simulink library "ECEF2LLA"  (R2018b)
settings: Solver=VariableStepAuto  StartTime=0.0  StopTime=10.0  RelTol=1e-3
settings Model: Creator=BI28030  LastModifiedBy=BI28030

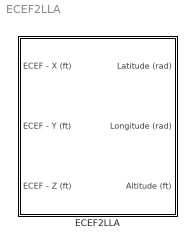
== system ECEF2LLA ==
  ECEF2LLA : Subsystem  mask{a=6378137, b=6356752.31424518}
      mask prompts: a "Semi-major axis (meters)"; b "Semi-major axis (meters)"

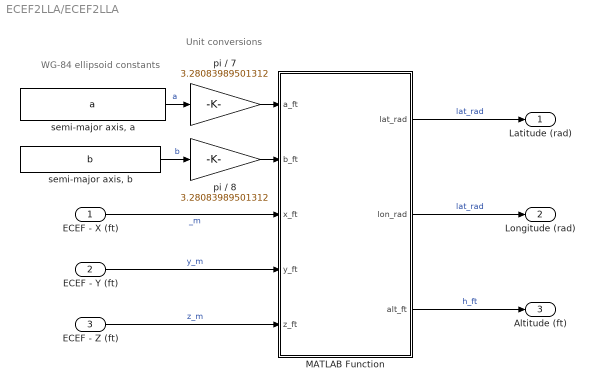
== system ECEF2LLA/ECEF2LLA ==
  note: WG-84 ellipsoid constants
  note: Unit conversions
  ECEF - X (ft) : Inport
  ECEF - Y (ft) : Inport  Port=2
  ECEF - Z (ft) : Inport  Port=3
  MATLAB Function : MATLAB Function  TreatAsAtomicUnit=on
  pi / 7 : Gain  Gain=3.28083989501312
  pi / 8 : Gain  Gain=3.28083989501312
  "semi-major axis, a" : Constant  Value=a
  "semi-major axis, b" : Constant  Value=b
  Latitude (rad) : Outport
  Longitude (rad) : Outport  Port=2
  Altitude (ft) : Outport  Port=3
  wires:
  pi / 8/1 -> MATLAB Function/2(b_ft)
  pi / 7/1 -> MATLAB Function/1(a_ft)
  ECEF - Z (ft)/1 -> MATLAB Function/5(z_ft)  "z_m"
  ECEF - Y (ft)/1 -> MATLAB Function/4(y_ft)  "y_m"
  ECEF - X (ft)/1 -> MATLAB Function/3(x_ft)  "_m"
  "semi-major axis, b"/1 -> pi / 8/1  "b"
  "semi-major axis, a"/1 -> pi / 7/1  "a"
  MATLAB Function/3(alt_ft) -> Altitude (ft)/1  "h_ft"
  MATLAB Function/1(lat_rad) -> Latitude (rad)/1  "lat_rad"
  MATLAB Function/2(lon_rad) -> Longitude (rad)/1  "lat_rad"

== matlab function ECEF2LLA/MATLAB Function ==
  data: a_ft input; b_ft input; x_ft input; y_ft input; z_ft input; lat_rad output; lon_rad output; alt_ft output
function [lat_rad,lon_rad,alt_ft] = ecef2lla(a_ft,b_ft,x_ft,y_ft,z_ft)
%#codegen

% Auxiliary values
p = hypot(x_ft,y_ft);
theta = atan((z_ft*a_ft) / (p*b_ft));

% Eccentricity
e1 = sqrt((a_ft^2-b_ft^2)/a_ft^2); % First eccentricity 
e2 = sqrt((a_ft^2-b_ft^2)/b_ft^2); % Second eccentricity

% Convert lat-lon
lat_rad = atan((z_ft + e2^2 * b_ft * sin(theta)^3) / (p - e1^2 * a_ft * cos(theta)^3));
lon_rad = atan(y_ft/x_ft);

% Ellipsoidal "radius"
N = a_ft./sqrt(1-(e1^2).*sin(lat_rad).^2);

% Convert altitude
alt_ft = (p / cos(lat_rad)) - N;
